simulink model "motor"  (R2024b)
settings: Solver=VariableStepAuto  StartTime=0.0  StopTime=2  RelTol=1e-3
settings Model: Creator=Austinchao  LastModifiedBy=Austinchao

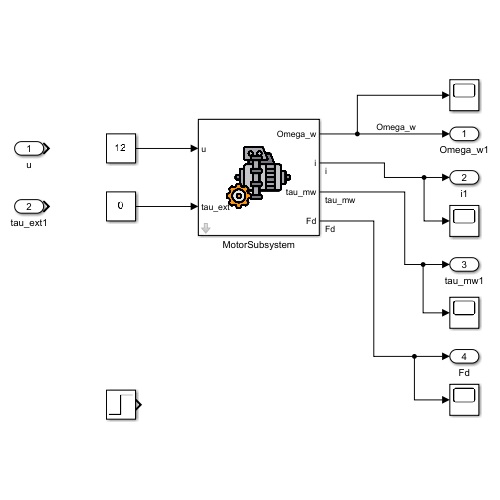
[thumbnail: Simulink's stored preview of the top-level diagram]
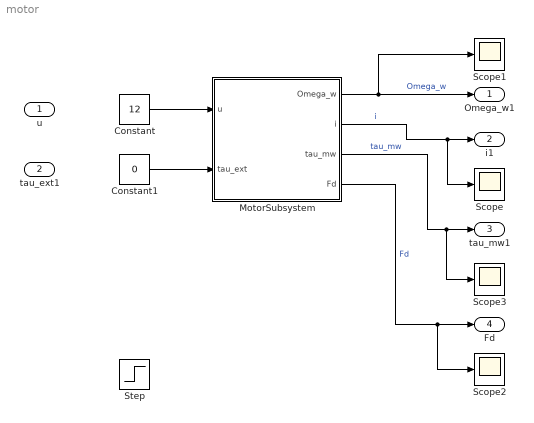
== system motor ==
  u : Inport
  tau_ext1 : Inport  Port=2
  Constant : Constant  Value=12
  Constant1 : Constant  Value=0
  MotorSubsystem : Subsystem  mask{Ra=3.75, Kt=0.013, Ke=0.013, n=90, Rw=0.04, Jm=1*10^-5, Jw=1*10^-4, Bm=3.95*10^-7, tau_c=0, dz=0, Ts=0, Bw=0}
      mask init:
      | Jeq = Jw + n^2 * Jm;
      | Beq = Bw + n^2 * Bm;
      | 
      | invRa = 1 / Ra;
      | nKt   = n * Kt;
      | invJeq= 1 / Jeq;
      | invRw = 1 / Rw;
      | Ke_n  = Ke * n;
      | 
      | alpha = n*Kt / (Ra*Rw);
      | beta  = n^2 * Kt * Ke / (Ra*Rw);
      | 
      | assert(Ra>0 && Rw>0 && n>0 && Jeq>0, 'Check Ra,Rw,n,Jm/Jw: must be >0');
      | assert(Kt>0 && Ke>0, 'Kt, Ke must be >0');
      | assert(Bm>=0 && Bw>=0, 'Bm,Bw must be >=0');
      | if exist('dz','var') && dz<0, dz = 0; end
      mask Display: image('models/icon/motor_icon.png', [0,0,0,0,60,60]);
  Scope{,1..3} (4 alike) : Scope
  Step : Step  Time=0.3  After=1.872  SampleTime=0
  Omega_w1 : Outport
  i1 : Outport  Port=2
  tau_mw1 : Outport  Port=3
  Fd : Outport  Port=4
  wires:
  MotorSubsystem/1(Omega_w) -> Omega_w1/1, Scope1/1  "Omega_w"
  MotorSubsystem/2(i) -> Scope/1, i1/1  "i"
  MotorSubsystem/4(Fd) -> Scope2/1, Fd/1  "Fd"
  MotorSubsystem/3(tau_mw) -> Scope3/1, tau_mw1/1  "tau_mw"
  Constant/1 -> MotorSubsystem/1(u)
  Constant1/1 -> MotorSubsystem/2(tau_ext)

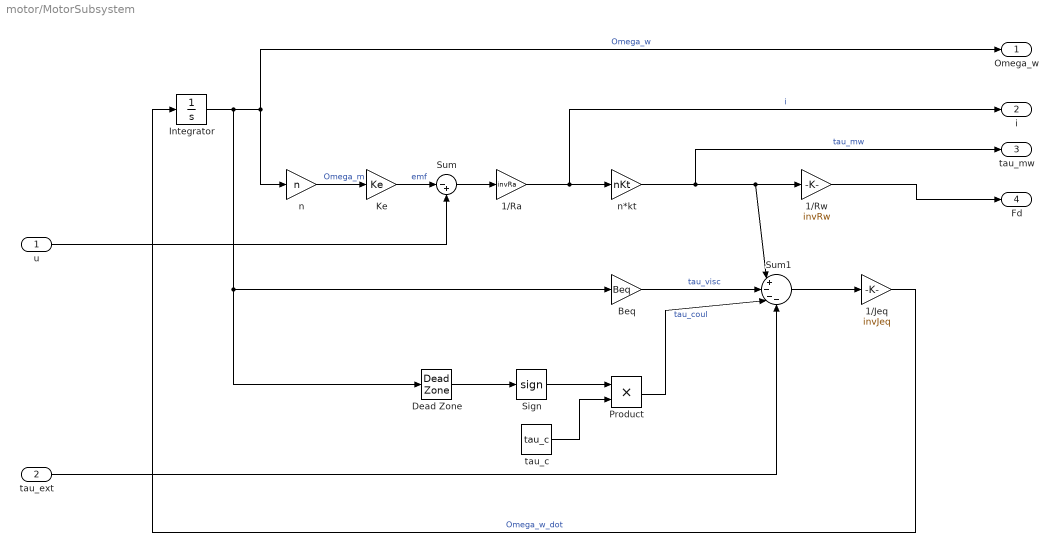
== system motor/MotorSubsystem ==
  u : Inport
  tau_ext : Inport  Port=2
  1/Jeq : Gain  Gain=invJeq
  1/Ra : Gain  Gain=invRa
  1/Rw : Gain  Gain=invRw
  Beq : Gain  Gain=Beq
  Dead Zone : DeadZone  LowerValue=-dz  UpperValue=dz
  Integrator : Integrator
  Ke : Gain  Gain=Ke
  Product : Product
  Sign : Signum
  Sum : Sum  Inputs=|-+
  Sum1 : Sum  Inputs=|+---
  n : Gain  Gain=n
  n*kt : Gain  Gain=nKt
  tau_c : Constant  Value=tau_c
  Omega_w : Outport
  i : Outport  Port=2
  tau_mw : Outport  Port=3
  Fd : Outport  Port=4
  wires:
  Sign/1 -> Product/1
  Integrator/1 -> Dead Zone/1, Beq/1, Omega_w/1, n/1  "Omega_w"
  n*kt/1 -> tau_mw/1, Sum1/1, 1/Rw/1  "tau_mw"
  Sum1/1 -> 1/Jeq/1
  Product/1 -> Sum1/3  "tau_coul"
  Dead Zone/1 -> Sign/1
  tau_c/1 -> Product/2
  1/Ra/1 -> i/1, n*kt/1  "i"
  n/1 -> Ke/1  "Omega_m"
  Ke/1 -> Sum/1  "emf"
  Beq/1 -> Sum1/2  "tau_visc"
  Sum/1 -> 1/Ra/1
  1/Jeq/1 -> Integrator/1  "Omega_w_dot"
  u/1 -> Sum/2
  1/Rw/1 -> Fd/1
  tau_ext/1 -> Sum1/4
